simulink model "Wersja_z_10_01"  (R2018b)
settings: Solver=ode23s  StartTime=0.0  StopTime=11  MaxStep=0.01  RelTol=1e-06  AbsTol=1e-06
values from neighbouring files (symbols this model uses):
  Cpas = 0.18    [Inity.m]
  Cpat = 3.8    [Inity.m]
  Cpvn = 20.5    [Inity.m]
  Csas = 0.08    [Inity.m]
  Csat = 1.6    [Inity.m]
  Csvn = 20.5    [Inity.m]
  Lpas = 0.000052    (= 5.2e-05)    [Inity.m]
  Lpat = 0.0017    [Inity.m]
  Lsas = 0.000062    (= 6.2e-05)    [Inity.m]
  Lsat = 0.0017    [Inity.m]
  Rpar = 0.05    [Inity.m]
  Rpas = 0.002    [Inity.m]
  Rpat = 0.01    [Inity.m]
  Rpcp = 0.25    [Inity.m]
  Rpvn = 0.006    [Inity.m]
  Rsar = 0.5    [Inity.m]
  Rsas = 0.003    [Inity.m]
  Rsat = 0.05    [Inity.m]
  Rscp = 0.52    [Inity.m]
  Rsvn = 0.075    [Inity.m]
settings Model: Creator=bartk  LastModifiedBy=bartk
settings SolverCC: AutoScaleAbsTol=off
settings DataIOCC: SaveFormat=Array
settings OptimizationCC: LifeSpan=inf
settings DebuggingCC: AlgebraicLoopMsg=none  SolverPrmCheckMsg=warning  StateNameClashWarn=warning
settings ModelReferenceCC: PropagateSignalLabelsOutOfModel=off
settings CodeAppCC: StateflowObjectComments=on

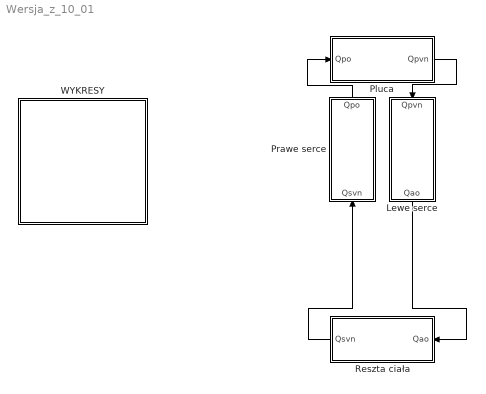
== system Wersja_z_10_01 ==
  "Lewe serce " : Subsystem
  "Pluca " : Subsystem
  "Prawe serce " : Subsystem
  "Reszta ciała " : Subsystem
  WYKRESY : Subsystem
  wires:
  "Reszta ciała "/1(Qsvn) -> "Prawe serce "/1(Qsvn)
  "Prawe serce "/1(Qpo) -> "Pluca "/1(Qpo)
  "Lewe serce "/1(Qao) -> "Reszta ciała "/1(Qao)
  "Pluca "/1(Qpvn) -> "Lewe serce "/1(Qpvn)

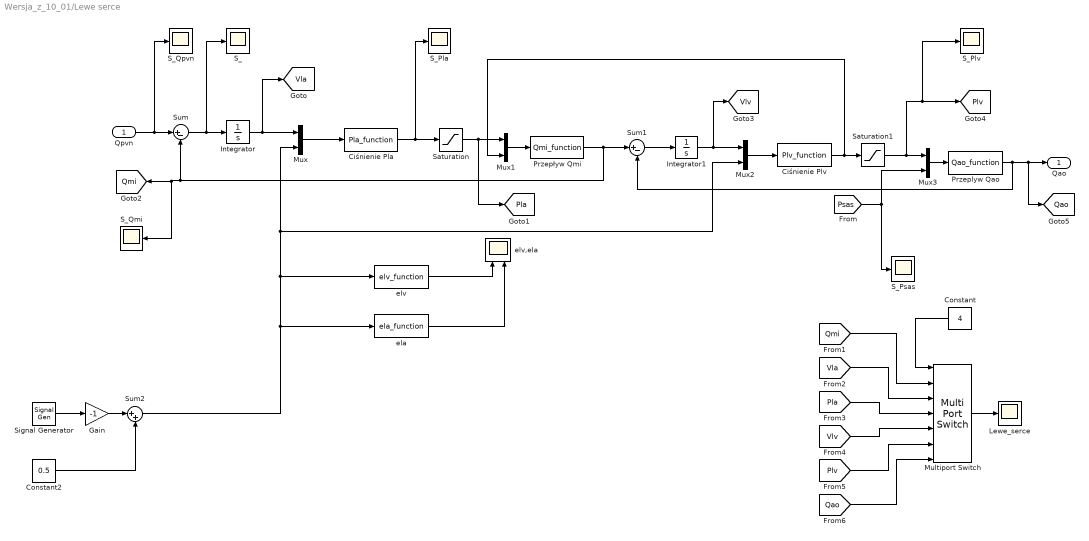
== system Wersja_z_10_01/Lewe serce  ==
  Qpvn : Inport
  Ciśnienie Pla : MATLABFcn  MATLABFcn=Pla_function
  "Ciśnienie Plv " : MATLABFcn  MATLABFcn=Plv_function
  Constant : Constant  Value=4
  Constant2 : Constant  Value=0.5
  Gain : Gain  Gain=-1
  Integrator : Integrator  InitialCondition=4
  Integrator1 : Integrator  InitialCondition=500
  Lewe_serce : Scope
  Multiport Switch : MultiPortSwitch  Inputs=6  OutMin=[1]  OutMax=[6]
  Mux{,1..3} (4 alike) : Mux  Inputs=2
  Przeplyw Qao : MATLABFcn  MATLABFcn=Qao_function
  Przepływ Qmi : MATLABFcn  MATLABFcn=Qmi_function
  S_ : Scope
  S_Pla : Scope
  S_Plv : Scope
  S_Psas : Scope
  S_Qmi : Scope
  S_Qpvn : Scope
  Saturation : Saturate  UpperLimit=inf  LowerLimit=0
  Saturation1 : Saturate  UpperLimit=inf  LowerLimit=0
  Signal Generator : SignalGenerator  WaveForm=sawtooth  Amplitude=0.5
  Sum : Sum  Inputs=|+-
  Sum1 : Sum  Inputs=|+-
  Sum2 : Sum  Inputs=|++
  ela : MATLABFcn  MATLABFcn=ela_function
  elv : MATLABFcn  MATLABFcn=elv_function
  elv,ela : Scope  NumInputPorts=2
  Qao : Outport
  tag scope: Pla=global, Plv=global, Qao=global, Qmi=global, Vla=global, Vlv=global
  wires:
  Przepływ Qmi/1 -> Sum1/1, S_Qmi/1, [Qmi], Sum/2
  Integrator1/1 -> Mux2/1, [Vlv]
  Sum2/1 -> ela/1, elv/1, Mux2/2, Mux/2
  Mux2/1 -> "Ciśnienie Plv "/1
  Mux3/1 -> Przeplyw Qao/1
  Przeplyw Qao/1 -> [Qao], Qao/1, Sum1/2
  Sum1/1 -> Integrator1/1
  [Psas] -> Mux3/2, S_Psas/1
  "Ciśnienie Plv "/1 -> Saturation1/1, Mux1/2
  Ciśnienie Pla/1 -> Saturation/1, S_Pla/1
  Mux1/1 -> Przepływ Qmi/1
  Mux/1 -> Ciśnienie Pla/1
  Integrator/1 -> Mux/1, [Vla]
  Sum/1 -> S_/1, Integrator/1
  Saturation/1 -> Mux1/1, [Pla]
  Qpvn/1 -> S_Qpvn/1, Sum/1
  elv/1 -> elv,ela/1
  ela/1 -> elv,ela/2
  [Qmi] -> Multiport Switch/2
  [Pla] -> Multiport Switch/4
  [Qao] -> Multiport Switch/7
  Multiport Switch/1 -> Lewe_serce/1
  [Plv] -> Multiport Switch/6
  Constant/1 -> Multiport Switch/1
  [Vla] -> Multiport Switch/3
  [Vlv] -> Multiport Switch/5
  Gain/1 -> Sum2/1
  Constant2/1 -> Sum2/2
  Signal Generator/1 -> Gain/1
  Saturation1/1 -> Mux3/1, S_Plv/1, [Plv]

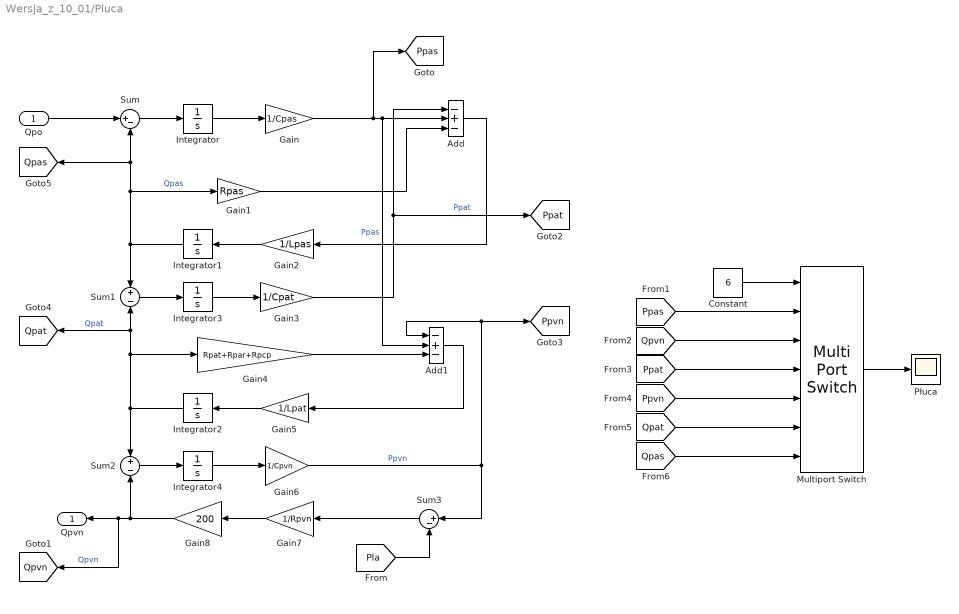
== system Wersja_z_10_01/Pluca  ==
  Qpo : Inport
  Add : Sum  Inputs=-+-
  Add1 : Sum  Inputs=-+-
  Constant : Constant  Value=6
  Gain : Gain  Gain=1/Cpas
  Gain1 : Gain  Gain=Rpas
  Gain2 : Gain  Gain=1/Lpas
  Gain3 : Gain  Gain=1/Cpat
  Gain4 : Gain  Gain=Rpat+Rpar+Rpcp
  Gain5 : Gain  Gain=1/Lpat
  Gain6 : Gain  Gain=1/Cpvn
  Gain7 : Gain  Gain=1/Rpvn
  Gain8 : Gain  Gain=200
  Integrator : Integrator  InitialCondition=30
  Integrator1 : Integrator
  Integrator2 : Integrator
  Integrator3 : Integrator  InitialCondition=30
  Integrator4 : Integrator  InitialCondition=8
  Multiport Switch : MultiPortSwitch  Inputs=6  OutMin=[1]  OutMax=[6]
  Płuca : Scope
  Sum : Sum  Inputs=|+-
  Sum1 : Sum  Inputs=+-
  Sum2 : Sum  Inputs=+-
  Sum3 : Sum  Inputs=|+-
  Qpvn : Outport
  tag scope: Ppas=global, Ppat=global, Ppvn=global, Qpas=global, Qpat=global, Qpvn=global
  wires:
  Gain6/1 -> [Ppvn], Add1/1, Sum3/1  "Ppvn"
  [Pla] -> Sum3/2
  Sum2/1 -> Integrator4/1
  Gain3/1 -> Add/1, [Ppat]  "Ppat"
  Integrator/1 -> Gain/1
  Add/1 -> Gain2/1
  Add1/1 -> Gain5/1
  Gain4/1 -> Add1/3
  Sum1/1 -> Integrator3/1
  Sum/1 -> Integrator/1
  Qpo/1 -> Sum/1
  Sum3/1 -> Gain7/1
  Gain1/1 -> Add/3
  Gain5/1 -> Integrator2/1
  Gain2/1 -> Integrator1/1
  Integrator3/1 -> Gain3/1
  Integrator4/1 -> Gain6/1
  [Ppas] -> Multiport Switch/2
  Multiport Switch/1 -> Płuca/1
  Constant/1 -> Multiport Switch/1
  [Qpvn] -> Multiport Switch/3
  Gain7/1 -> Gain8/1
  [Ppat] -> Multiport Switch/4
  [Ppvn] -> Multiport Switch/5
  [Qpat] -> Multiport Switch/6
  [Qpas] -> Multiport Switch/7
  Gain8/1 -> [Qpvn], Qpvn/1, Sum2/2  "Qpvn"
  Integrator1/1 -> [Qpas], Sum/2, Gain1/1, Sum1/1  "Qpas"
  Integrator2/1 -> Gain4/1, [Qpat], Sum1/2, Sum2/1  "Qpat"
  Gain/1 -> [Ppas], Add1/2, Add/2  "Ppas"

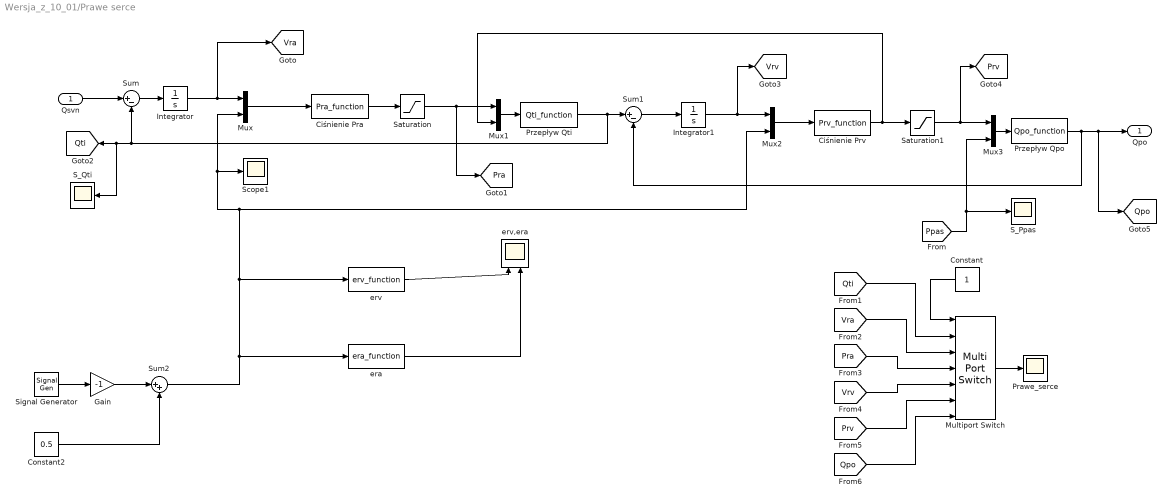
== system Wersja_z_10_01/Prawe serce  ==
  Qsvn : Inport
  "Ciśnienie Pra " : MATLABFcn  MATLABFcn=Pra_function
  Ciśnienie Prv : MATLABFcn  MATLABFcn=Prv_function
  Constant : Constant
  Constant2 : Constant  Value=0.5
  Gain : Gain  Gain=-1
  Integrator : Integrator  InitialCondition=4
  Integrator1 : Integrator  InitialCondition=400
  Multiport Switch : MultiPortSwitch  Inputs=6  OutMin=[1]  OutMax=[6]
  Mux{,1..3} (4 alike) : Mux  Inputs=2
  Prawe_serce : Scope
  Przepływ Qpo : MATLABFcn  MATLABFcn=Qpo_function
  Przepływ Qti : MATLABFcn  MATLABFcn=Qti_function
  S_Ppas : Scope
  S_Qti : Scope
  Saturation : Saturate  UpperLimit=inf  LowerLimit=0  LinearizeAsGain=off
  Saturation1 : Saturate  UpperLimit=inf  LowerLimit=0
  Scope1 : Scope
  Signal Generator : SignalGenerator  WaveForm=sawtooth  Amplitude=0.5
  Sum : Sum  Inputs=|+-
  Sum1 : Sum  Inputs=|+-
  Sum2 : Sum  Inputs=|++
  era : MATLABFcn  MATLABFcn=era_function
  erv : MATLABFcn  MATLABFcn=erv_function
  erv,era : Scope  NumInputPorts=2
  Qpo : Outport
  tag scope: Pra=global, Prv=global, Qpo=global, Qti=global, Vra=global, Vrv=global
  wires:
  Qsvn/1 -> Sum/1
  Sum/1 -> Integrator/1
  Integrator/1 -> Mux/1, [Vra]
  Mux/1 -> "Ciśnienie Pra "/1
  "Ciśnienie Pra "/1 -> Saturation/1
  Mux1/1 -> Przepływ Qti/1
  Przepływ Qti/1 -> Sum1/1, S_Qti/1, [Qti], Sum/2
  Sum1/1 -> Integrator1/1
  Integrator1/1 -> Mux2/1, [Vrv]
  Mux2/1 -> Ciśnienie Prv/1
  Ciśnienie Prv/1 -> Saturation1/1, Mux1/2
  [Ppas] -> Mux3/2, S_Ppas/1
  Mux3/1 -> Przepływ Qpo/1
  Przepływ Qpo/1 -> Qpo/1, [Qpo], Sum1/2
  Sum2/1 -> era/1, erv/1, Mux2/2, Mux/2, Scope1/1
  Saturation/1 -> Mux1/1, [Pra]
  Saturation1/1 -> [Prv], Mux3/1
  erv/1 -> erv,era/1
  era/1 -> erv,era/2
  Multiport Switch/1 -> Prawe_serce/1
  [Pra] -> Multiport Switch/4
  [Qpo] -> Multiport Switch/7
  [Prv] -> Multiport Switch/6
  [Vrv] -> Multiport Switch/5
  [Vra] -> Multiport Switch/3
  [Qti] -> Multiport Switch/2
  Constant/1 -> Multiport Switch/1
  Gain/1 -> Sum2/1
  Constant2/1 -> Sum2/2
  Signal Generator/1 -> Gain/1

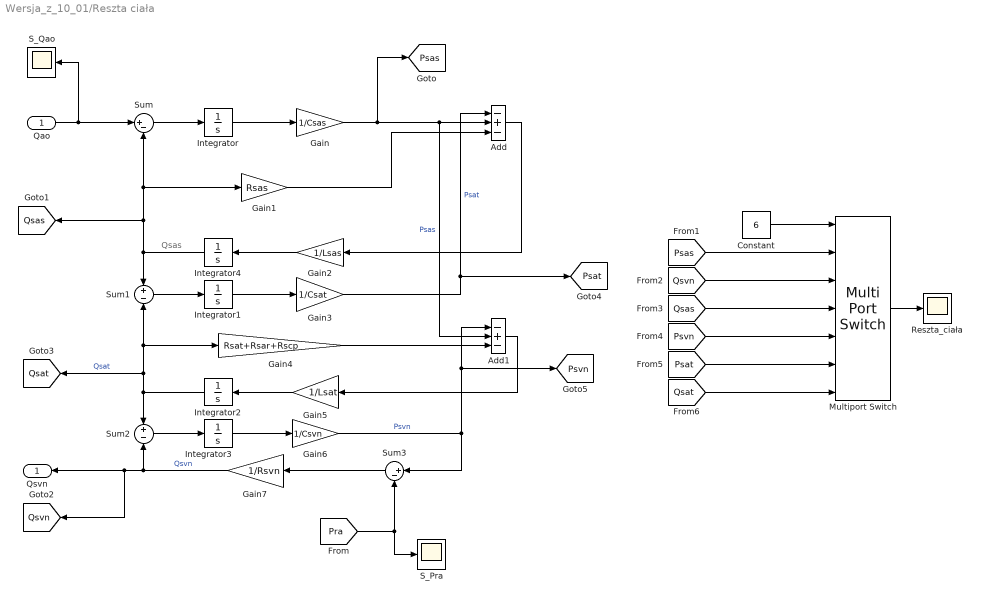
== system Wersja_z_10_01/Reszta ciała  ==
  note: Qsas
  Qao : Inport
  Add : Sum  Inputs=-+-
  Add1 : Sum  Inputs=-+-
  Constant : Constant  Value=6
  Gain : Gain  Gain=1/Csas
  Gain1 : Gain  Gain=Rsas
  Gain2 : Gain  Gain=1/Lsas
  Gain3 : Gain  Gain=1/Csat
  Gain4 : Gain  Gain=Rsat+Rsar+Rscp
  Gain5 : Gain  Gain=1/Lsat
  Gain6 : Gain  Gain=1/Csvn
  Gain7 : Gain  Gain=1/Rsvn
  Integrator : Integrator  InitialCondition=100
  Integrator1 : Integrator  InitialCondition=100
  Integrator2 : Integrator
  Integrator3 : Integrator  InitialCondition=4
  Integrator4 : Integrator
  Multiport Switch : MultiPortSwitch  Inputs=6  OutMin=[1]  OutMax=[6]
  Reszta_ciała : Scope
  S_Pra : Scope
  S_Qao : Scope
  Sum : Sum  Inputs=|+-
  Sum1 : Sum  Inputs=+-
  Sum2 : Sum  Inputs=+-
  Sum3 : Sum  Inputs=|+-
  Qsvn : Outport
  tag scope: Psas=global, Psat=global, Psvn=global, Qsas=global, Qsat=global, Qsvn=global
  wires:
  Qao/1 -> Sum/1, S_Qao/1
  Sum/1 -> Integrator/1
  Integrator/1 -> Gain/1
  Gain/1 -> [Psas], Add1/2, Add/2  "Psas"
  Gain1/1 -> Add/3
  Add/1 -> Gain2/1
  Sum1/1 -> Integrator1/1
  Gain3/1 -> [Psat], Add/1  "Psat"
  Gain4/1 -> Add1/3
  Add1/1 -> Gain5/1
  Sum2/1 -> Integrator3/1
  Gain6/1 -> Sum3/1, [Psvn], Add1/1  "Psvn"
  Sum3/1 -> Gain7/1
  Gain7/1 -> [Qsvn], Qsvn/1, Sum2/2  "Qsvn"
  [Pra] -> Sum3/2, S_Pra/1
  Integrator3/1 -> Gain6/1
  Integrator1/1 -> Gain3/1
  Gain2/1 -> Integrator4/1
  Gain5/1 -> Integrator2/1
  [Qsvn] -> Multiport Switch/3
  Constant/1 -> Multiport Switch/1
  Multiport Switch/1 -> Reszta_ciała/1
  [Psas] -> Multiport Switch/2
  [Qsas] -> Multiport Switch/4
  [Psvn] -> Multiport Switch/5
  [Psat] -> Multiport Switch/6
  [Qsat] -> Multiport Switch/7
  Integrator4/1 -> Sum/2, Gain1/1, [Qsas], Sum1/1
  Integrator2/1 -> Gain4/1, Sum1/2, [Qsat], Sum2/1  "Qsat"

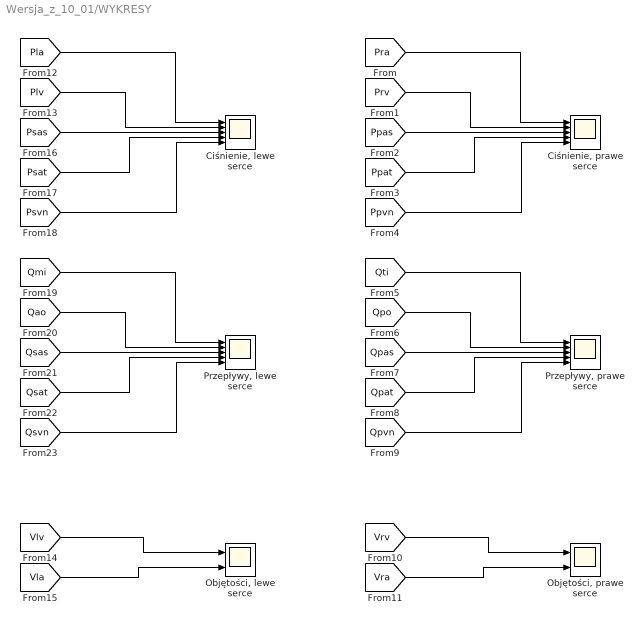
== system Wersja_z_10_01/WYKRESY ==
  "Ciśnienie, lewe serce" : Scope  NumInputPorts=5
  "Ciśnienie, prawe serce" : Scope  NumInputPorts=5
  "Objętości, lewe serce" : Scope  NumInputPorts=2
  "Objętości, prawe serce" : Scope  NumInputPorts=2
  "Przepływy, lewe serce" : Scope  NumInputPorts=5
  "Przepływy, prawe serce" : Scope  NumInputPorts=5
  wires:
  [Pra] -> "Ciśnienie, prawe serce"/1
  [Prv] -> "Ciśnienie, prawe serce"/2
  [Ppas] -> "Ciśnienie, prawe serce"/3
  [Ppat] -> "Ciśnienie, prawe serce"/4
  [Ppvn] -> "Ciśnienie, prawe serce"/5
  [Qpvn] -> "Przepływy, prawe serce"/5
  [Qpat] -> "Przepływy, prawe serce"/4
  [Qpo] -> "Przepływy, prawe serce"/2
  [Qti] -> "Przepływy, prawe serce"/1
  [Qpas] -> "Przepływy, prawe serce"/3
  [Vrv] -> "Objętości, prawe serce"/1
  [Vra] -> "Objętości, prawe serce"/2
  [Psvn] -> "Ciśnienie, lewe serce"/5
  [Vlv] -> "Objętości, lewe serce"/1
  [Vla] -> "Objętości, lewe serce"/2
  [Pla] -> "Ciśnienie, lewe serce"/1
  [Qmi] -> "Przepływy, lewe serce"/1
  [Plv] -> "Ciśnienie, lewe serce"/2
  [Qsas] -> "Przepływy, lewe serce"/3
  [Qao] -> "Przepływy, lewe serce"/2
  [Psas] -> "Ciśnienie, lewe serce"/3
  [Qsvn] -> "Przepływy, lewe serce"/5
  [Qsat] -> "Przepływy, lewe serce"/4
  [Psat] -> "Ciśnienie, lewe serce"/4
